simulink model "simulation2024a"  (R2024a)
settings: Solver=ode4  StartTime=0.0  StopTime=20  FixedStep=0.01  RelTol=1e-3
values from neighbouring files (symbols this model uses):
  Eta_initial = [0;0;0]    [Feb21_tutorial.m]    (also in model.m; tutorial.m)
  V_initial = [0;0;0]    [Feb21_tutorial.m]    (also in model.m = [0;0;0]+[EN.current_speed';0]; tutorial.m)
undefined symbols (not defined in the file or in its folder): DC, DCon, TN
libraries: slpidlib x1
settings Model: Creator=Irene  LastModifiedBy=SCK

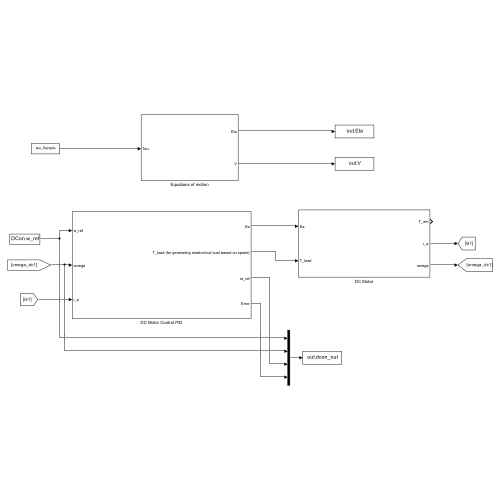
[thumbnail: Simulink's stored preview of the top-level diagram]
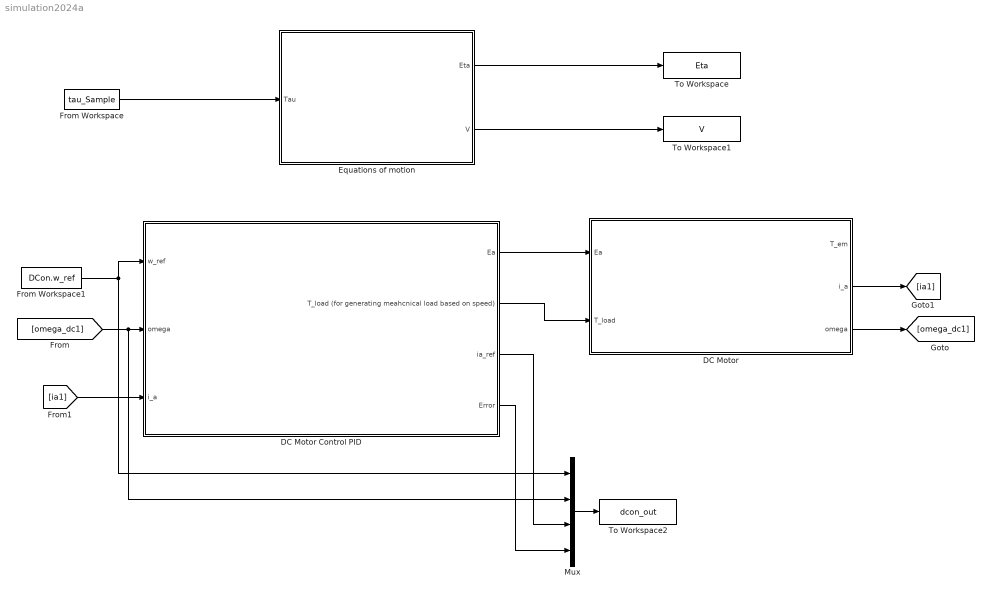
== system simulation2024a ==
  DC Motor : Subsystem
  DC Motor Control PID : Subsystem
  Equations of motion : Subsystem
  From Workspace : FromWorkspace  VariableName=tau_Sample
  From Workspace1 : FromWorkspace  VariableName=DCon.w_ref
  Mux : Mux
  To Workspace : ToWorkspace  VariableName=Eta  SampleTime=-1
  To Workspace1 : ToWorkspace  VariableName=V  SampleTime=-1
  To Workspace2 : ToWorkspace  VariableName=dcon_out  SampleTime=-1
  wires:
  From Workspace/1 -> Equations of motion/1(Tau)
  Equations of motion/1(Eta) -> To Workspace/1
  Equations of motion/2(V) -> To Workspace1/1
  DC Motor/3(omega) -> [omega_dc1]
  DC Motor/2(i_a) -> [ia1]
  From Workspace1/1 -> Mux/1, DC Motor Control PID/1(w_ref)
  [omega_dc1] -> Mux/2, DC Motor Control PID/2(omega)
  DC Motor Control PID/3(ia_ref) -> Mux/3
  DC Motor Control PID/4(Error) -> Mux/4
  Mux/1 -> To Workspace2/1
  DC Motor Control PID/1(Ea) -> DC Motor/1(Ea)
  DC Motor Control PID/2(T_load (for generating meahcnical load based on speed)) -> DC Motor/2(T_load)
  [ia1] -> DC Motor Control PID/3(i_a)

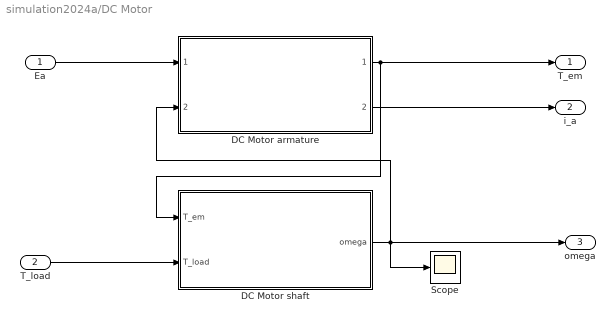
== system simulation2024a/DC Motor ==
  Ea : Inport
  T_load : Inport  Port=2
  DC Motor armature : Subsystem  ReferencedSubsystem=DC_Motor_armature
  DC Motor shaft : Subsystem
  Scope : Scope
  T_em : Outport
  i_a : Outport  Port=2
  omega : Outport  Port=3
  wires:
  DC Motor armature/1 -> T_em/1, DC Motor shaft/1(T_em)
  DC Motor shaft/1(omega) -> omega/1, Scope/1, DC Motor armature/2
  Ea/1 -> DC Motor armature/1
  T_load/1 -> DC Motor shaft/2(T_load)
  DC Motor armature/2 -> i_a/1

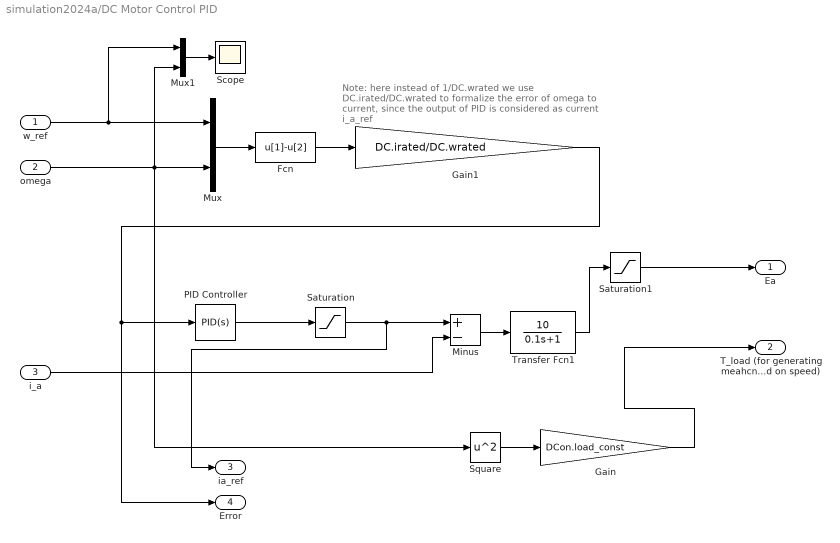
== system simulation2024a/DC Motor Control PID ==
  note: Note: here instead of 1/DC.wrated we use DC.irated/DC.wrated to formalize the error of omega to current, since the output of PID is considered as current i_a_ref
  w_ref : Inport
  omega : Inport  Port=2
  i_a : Inport  Port=3
  Fcn : Fcn  Expr=u[1]-u[2]
  Gain : Gain  Gain=DCon.load_const
  Gain1 : Gain  Gain=DC.irated/DC.wrated
  Minus : Sum  Inputs=+-
  Mux : Mux  Inputs=2
  Mux1 : Mux  Inputs=2
  PID Controller : slpidlib/PID Controller  Controller=PID  Form=Parallel  TimeDomain=Continuous-time  UseExternalTs=off  SampleTime=-1  IntegratorMethod=Forward Euler  FilterMethod=Forward Euler  ControllerParametersSource=internal  P=DCon.Kp  I=DCon.Ki  UseKiTs=off  D=DCon.Kd  UseExternalDerivativeSource=off  N=DCon.N  UseFilter=on  TunerSelectOption=Transfer Function Based (PID Tuner App)  InitialConditionSource=internal  InitialConditionForIntegrator=0  InitialConditionForFilter=0  DifferentiatorICPrevScaledInput=0  ExternalReset=none  TrackingMode=off  Kt=1  LimitOutput=off  SatLimitsSource=internal  UpperSaturationLimit=inf  LowerSaturationLimit=-inf  LinearizeAsGain=on  AntiWindupMode=none  Kb=1  LimitIntegrator=off  UpperIntegratorSaturationLimit=inf  LowerIntegratorSaturationLimit=-inf  POutMin=[]  POutMax=[]  IOutMin=[]  IOutMax=[]  DOutMin=[]  DOutMax=[]  NOutMin=[]  NOutMax=[]  SumOutMin=[]  SumOutMax=[]  SaturationOutMin=[]  SaturationOutMax=[]  PParamMin=[]  PParamMax=[]  IParamMin=[]  IParamMax=[]  DParamMin=[]  DParamMax=[]  NParamMin=[]  NParamMax=[]  KbParamMin=[]  KbParamMax=[]  KtParamMin=[]  KtParamMax=[]  KbOutMin=[]  KbOutMax=[]  KtOutMin=[]  KtOutMax=[]  IntegratorOutMin=[]  IntegratorOutMax=[]  FilterOutMin=[]  FilterOutMax=[]  SumI1OutMin=[]  SumI1OutMax=[]  SumI2OutMin=[]  SumI2OutMax=[]  SumI3OutMin=[]  SumI3OutMax=[]  SumI4OutMin=[]  SumI4OutMax=[]  SumDOutMin=[]  SumDOutMax=[]  DifferentiatorOutMin=[]  DifferentiatorOutMax=[]  FilterDiffOutCoefMin=[]  FilterDiffOutCoefMax=[]  ReciprocalOutMin=[]  ReciprocalOutMax=[]  SumDenOutMin=[]  SumDenOutMax=[]  SumNumOutMin=[]  SumNumOutMax=[]  DivideOutMin=[]  DivideOutMax=[]  UdiffTsProdOutMin=[]  UdiffTsProdOutMax=[]  NTsProdOutMin=[]  NTsProdOutMax=[]  UintegralTsProdOutMin=[]  UintegralTsProdOutMax=[]  UngainTsProdOutMin=[]  UngainTsProdOutMax=[]  ClampingZeroOutDataTypeStr=Inherit: Inherit via back propagation  ClampingZeroOutMin=[]  ClampingZeroOutMax=[]  FilterDenConstantOutDataTypeStr=Inherit: Inherit via back propagation  FilterDenConstantOutMin=[]  FilterDenConstantOutMax=[]  PCopyOutDataTypeStr=Inherit: Inherit via back propagation  PCopyOutMin=[]  PCopyOutMax=[]  NCopyOutDataTypeStr=Inherit: Inherit via back propagation  NCopyOutMin=[]  NCopyOutMax=[]  IntegratorContinuousStateAttributes=''  IntegratorStateMustResolveToSignalObject=off  IntegratorRTWStateStorageClass=Auto  FilterContinuousStateAttributes=''  FilterStateMustResolveToSignalObject=off  FilterRTWStateStorageClass=Auto  ParallelPVariant=InternalParameters  IdealPVariant=Disabled  IVariant=InternalParameters  DVariant=InternalParameters  IntegratorVariant=Continuous  SatVariant=Disabled  AWVariant=Passthrough  PCopyVariant=Disabled  TRVariant=Disabled  FdbkBlocksVariant=Forward  IdealPFdbkVariant=Disabled  SatFdbkVariant=Disabled  DerivativeFilterVariant=ContFilter  NVariant=InternalParameters  NCopyVariant=Disabled  FilterICVariant=InternalICsFilter  IntegratorICVariant=InternalICs  ExternalResetVariant=Disabled  TRSumVariant=Passthrough  SumFdbkVariant=Disabled  SumVariant=Sum_PID  TsampFilterVariant=InternalTs  TsampNgainVariant=Passthrough  TsampIntegralVariant=Disabled_SignalSpec  ExternalSaturationOutDataTypeStr=Inherit: Same as second input  DerivativeSourceVariant=ErrorSignal
  Saturation : Saturate  UpperLimit=DC.irated  LowerLimit=-DC.irated
  Saturation1 : Saturate  UpperLimit=DC.vrated  LowerLimit=-DC.vrated
  Scope : Scope
  Square : Math  Operator=square
  Transfer Fcn1 : TransferFcn  Numerator=[10]  Denominator=[0.1 1]
  Ea : Outport
  T_load (for generating meahcnical load based on speed) : Outport  Port=2
  ia_ref : Outport  Port=3
  Error : Outport  Port=4
  wires:
  Transfer Fcn1/1 -> Saturation1/1
  i_a/1 -> Minus/2
  Minus/1 -> Transfer Fcn1/1
  Mux/1 -> Fcn/1
  Fcn/1 -> Gain1/1
  Square/1 -> Gain/1
  Saturation/1 -> ia_ref/1, Minus/1
  Gain1/1 -> Error/1, PID Controller/1
  PID Controller/1 -> Saturation/1
  Saturation1/1 -> Ea/1
  Gain/1 -> T_load (for generating meahcnical load based on speed)/1
  omega/1 -> Square/1, Mux1/2, Mux/2
  w_ref/1 -> Mux1/1, Mux/1
  Mux1/1 -> Scope/1

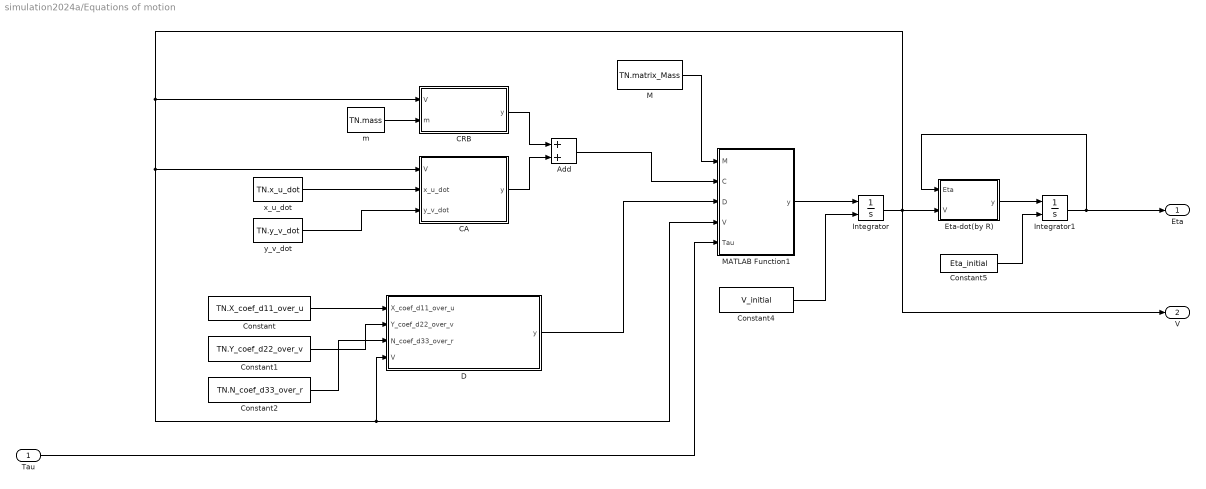
== system simulation2024a/Equations of motion ==
  Tau : Inport
  Add : Sum
  CA : MATLAB Function  TreatAsAtomicUnit=on
  CRB : MATLAB Function  TreatAsAtomicUnit=on
  Constant : Constant  Value=TN.X_coef_d11_over_u
  Constant1 : Constant  Value=TN.Y_coef_d22_over_v
  Constant2 : Constant  Value=TN.N_coef_d33_over_r
  Constant4 : Constant  Value=V_initial
  Constant5 : Constant  Value=Eta_initial
  D : MATLAB Function  TreatAsAtomicUnit=on
  Eta-dot(by R) : MATLAB Function  TreatAsAtomicUnit=on
  Integrator : Integrator  InitialConditionSource=external
  Integrator1 : Integrator  InitialConditionSource=external
  M : Constant  Value=TN.matrix_Mass
  MATLAB Function1 : MATLAB Function  TreatAsAtomicUnit=on
  m : Constant  Value=TN.mass
  "x_u_dot " : Constant  Value=TN.x_u_dot
  y_v_dot : Constant  Value=TN.y_v_dot
  Eta : Outport
  V : Outport  Port=2
  wires:
  Constant1/1 -> D/2(Y_coef_d22_over_v)
  m/1 -> CRB/2(m)
  Constant4/1 -> Integrator/2
  Integrator1/1 -> Eta/1, Eta-dot(by R)/1(Eta)
  "x_u_dot "/1 -> CA/2(x_u_dot)
  Integrator/1 -> V/1, Eta-dot(by R)/2(V), MATLAB Function1/4(V), D/4(V), CA/1(V), CRB/1(V)
  MATLAB Function1/1(y) -> Integrator/1
  Constant2/1 -> D/3(N_coef_d33_over_r)
  y_v_dot/1 -> CA/3(y_v_dot)
  Add/1 -> MATLAB Function1/2(C)
  Constant5/1 -> Integrator1/2
  D/1(y) -> MATLAB Function1/3(D)
  CA/1(y) -> Add/2
  Eta-dot(by R)/1(y) -> Integrator1/1
  M/1 -> MATLAB Function1/1(M)
  CRB/1(y) -> Add/1
  Constant/1 -> D/1(X_coef_d11_over_u)
  Tau/1 -> MATLAB Function1/5(Tau)

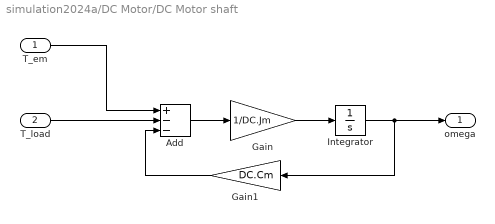
== system simulation2024a/DC Motor/DC Motor shaft ==
  T_em : Inport
  T_load : Inport  Port=2
  Add : Sum  Inputs=+--
  Gain : Gain  Gain=1/DC.Jm
  Gain1 : Gain  Gain=DC.Cm
  Integrator : Integrator
  omega : Outport
  wires:
  Gain/1 -> Integrator/1
  Add/1 -> Gain/1
  Integrator/1 -> omega/1, Gain1/1
  Gain1/1 -> Add/3
  T_em/1 -> Add/1
  T_load/1 -> Add/2

== matlab function simulation2024a/Equations of motion/CA ==
  data: V input; y output; x_u_dot input; y_v_dot input
function y = C_A(V,x_u_dot,y_v_dot)
a1=x_u_dot*V(1);
a2=y_v_dot*V(2);
y = [0   0   a2;
     0   0  -a1;
     -a2 a1  0];

== matlab function simulation2024a/Equations of motion/CRB ==
  data: V input; y output; m input
function y = C_RB(V,m)

y = [0       0      -m*V(2);
     0       0      m*V(1) ;
     m*V(2) -m*V(1) 0     ];

== matlab function simulation2024a/Equations of motion/MATLAB Function1 ==
  data: M input; C input; D input; V input; Tau input; y output
function y = motion_V_dot(M,C,D,V,Tau)

y = inv(M)*(Tau-C*V-D*V);

== matlab function simulation2024a/Equations of motion/D ==
  data: X_coef_d11_over_u input; y output; Y_coef_d22_over_v input; N_coef_d33_over_r input; V input
function y = D(X_coef_d11_over_u,Y_coef_d22_over_v,N_coef_d33_over_r,V)
d11=polyval(X_coef_d11_over_u,V(1));
d22=polyval(Y_coef_d22_over_v,V(2));
d33=polyval(N_coef_d33_over_r,V(3));
y = diag([d11 d22 d33]);

== matlab function simulation2024a/Equations of motion/Eta-dot(by R) ==
  data: Eta input; y output; V input
function y = Eta_dot(Eta,V)
psi=Eta(3);
R = [cos(psi) -sin(psi) 0;
     sin(psi)  cos(psi) 0;
      0        0        1];
y=R*V;
